simulink model "FORWARD_KINEMATICS"  (R2016a)
settings: Solver=VariableStepAuto  StartTime=0.0  StopTime=5  RelTol=1e-3
values from neighbouring files (symbols this model uses):
  l1 = 315    [FORWARD_KINEMATICS_DELTA_ROBOT.m]    (also in Inverse_Dynamic_Model.m = 0.315; Inverse_Dynamic_Model_Test_Result.m = 0.3; Kinematic_Dimension.m; _PARAMETER_OF_DELTA_ROBOT.m = 0.315)
  phi = [phi1; phi2; phi3]    [Inverse_Dynamic_Model.m]    (also in Inverse_Dynamic_Model_Test_Result.m; Kinematic_Dimension.m; _PARAMETER_OF_DELTA_ROBOT.m)
  r = r1- r2    (= 150)    [FORWARD_KINEMATICS_DELTA_ROBOT.m]    (also in Inverse_Dynamic_Model.m = -0.15; Inverse_Dynamic_Model_Test_Result.m = -0.15; Kinematic_Dimension.m; _PARAMETER_OF_DELTA_ROBOT.m = -0.15)
settings Model: Creator=computer  LastModifiedBy=ThanhUTC
settings DataIOCC: SaveFormat=Array

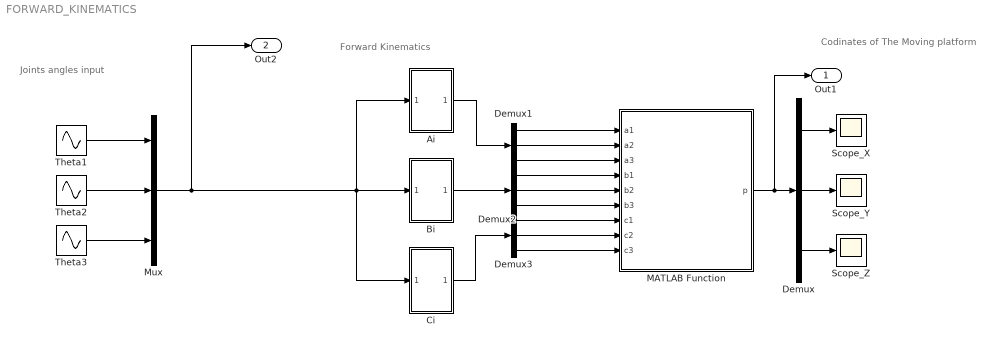
== system FORWARD_KINEMATICS ==
  note: Forward Kinematics
  note: Codinates of The Moving platform
  note: Joints angles input
  Ai : Subsystem
  Bi : Subsystem
  Ci : Subsystem
  Demux{,1..3} (4 alike) : Demux  Outputs=3
  MATLAB Function : MATLAB Function  TreatAsAtomicUnit=on
  Mux : Mux  Inputs=3
  Scope_X : Scope
  Scope_Y : Scope
  Scope_Z : Scope
  Theta1 : Sin  Frequency=1.5  SampleTime=0
  Theta2 : Sin  Amplitude=0.5  Bias=pi/8  Frequency=pi/2  SampleTime=0
  Theta3 : Sin  Amplitude=0.5  Frequency=pi  SampleTime=0
  Out1 : Outport
  Out2 : Outport  Port=2
  wires:
  Theta2/1 -> Mux/2
  Theta1/1 -> Mux/1
  Theta3/1 -> Mux/3
  Demux/3 -> Scope_Z/1
  Demux/2 -> Scope_Y/1
  Demux/1 -> Scope_X/1
  MATLAB Function/1(p) -> Out1/1, Demux/1
  Bi/1(Out1) -> Demux2/1
  Demux3/2 -> MATLAB Function/8(c2)
  Demux3/1 -> MATLAB Function/7(c1)
  Mux/1 -> Out2/1, Ci/1(In1), Ai/1(In1), Bi/1(In1)
  Demux3/3 -> MATLAB Function/9(c3)
  Demux2/1 -> MATLAB Function/4(b1)
  Demux2/3 -> MATLAB Function/6(b3)
  Ai/1(Out1) -> Demux1/1
  Demux2/2 -> MATLAB Function/5(b2)
  Ci/1(Out1) -> Demux3/1
  Demux1/2 -> MATLAB Function/2(a2)
  Demux1/1 -> MATLAB Function/1(a1)
  Demux1/3 -> MATLAB Function/3(a3)

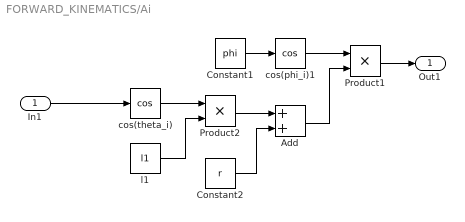
== system FORWARD_KINEMATICS/Ai ==
  In1 : Inport
  Add : Sum
  Constant1 : Constant  Value=phi
  Constant2 : Constant  Value=r
  Product1 : Product
  Product2 : Product
  cos(phi_i)1 : Trigonometry  Operator=cos
  cos(theta_i) : Trigonometry  Operator=cos
  l1 : Constant  Value=l1
  Out1 : Outport
  wires:
  Constant1/1 -> cos(phi_i)1/1
  cos(theta_i)/1 -> Product2/1
  In1/1 -> cos(theta_i)/1
  l1/1 -> Product2/2
  cos(phi_i)1/1 -> Product1/1
  Product2/1 -> Add/1
  Constant2/1 -> Add/2
  Add/1 -> Product1/2
  Product1/1 -> Out1/1

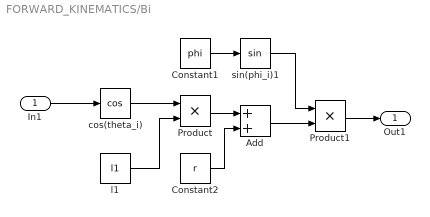
== system FORWARD_KINEMATICS/Bi ==
  In1 : Inport
  Add : Sum
  Constant1 : Constant  Value=phi
  Constant2 : Constant  Value=r
  Product : Product
  Product1 : Product
  cos(theta_i) : Trigonometry  Operator=cos
  l1 : Constant  Value=l1
  sin(phi_i)1 : Trigonometry
  Out1 : Outport
  wires:
  In1/1 -> cos(theta_i)/1
  l1/1 -> Product/2
  cos(theta_i)/1 -> Product/1
  Constant1/1 -> sin(phi_i)1/1
  Product/1 -> Add/1
  Constant2/1 -> Add/2
  Add/1 -> Product1/2
  sin(phi_i)1/1 -> Product1/1
  Product1/1 -> Out1/1

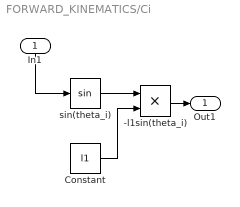
== system FORWARD_KINEMATICS/Ci ==
  In1 : Inport
  -l1sin(theta_i) : Product
  Constant : Constant  Value=l1
  sin(theta_i) : Trigonometry
  Out1 : Outport
  wires:
  Constant/1 -> -l1sin(theta_i)/2
  In1/1 -> sin(theta_i)/1
  -l1sin(theta_i)/1 -> Out1/1
  sin(theta_i)/1 -> -l1sin(theta_i)/1

== matlab function FORWARD_KINEMATICS/MATLAB Function ==
  data: p output; a1 input; a2 input; a3 input; b1 input; b2 input; b3 input; c1 input; c2 input; c3 input
function p = equasol(a1, a2, a3, b1, b2, b3, c1, c2, c3)
%#codegen
 coder.extrinsic('solequa'); 
 p = zeros(3,1);
 p = solequa(a1, a2, a3, b1, b2, b3, c1, c2, c3);
